simulink model "untitled"  (R2022a)
settings: Solver=FixedStepAuto  StartTime=0.0  StopTime=40  FixedStep=0.001768  RelTol=1e-3  EnableMultiTasking=on
values from neighbouring files (symbols this model uses):
  AlphacKhwgr = 0    [MELMNNSTRCECP.m]
  AlphavKhwgr = 0.914    [MELMNNSTRCECP.m]
  gr = 4    [MELMNNSTRCECP.m]
  JrC1 = 0.0675    [MELMNNSTRCECP.m]
  Khw = 5.81    [MELMNNSTRCECP.m]
libraries: dspstat3 x1, spsTriangleGeneratorLib x1
settings Model: Creator=dimas  LastModifiedBy=dimas
settings DataIOCC: SaveFormat=Array  ReturnWorkspaceOutputs=off
settings DebuggingCC: SolverPrmCheckMsg=warning  UnconnectedInputMsg=warning  UnconnectedOutputMsg=warning  UnconnectedLineMsg=warning  SFUnexpectedBacktrackingDiag=warning  SFNoUnconditionalDefaultTransitionDiag=warning  SFExecutionAtInitializationDiag=none  UnderSpecifiedDimensionMsg=warning
settings ModelReferenceCC: PropagateSignalLabelsOutOfModel=off
settings CodeAppCC: StateflowObjectComments=on
settings GRTTargetCC: TargetLangStandard=C89/C90 (ANSI)

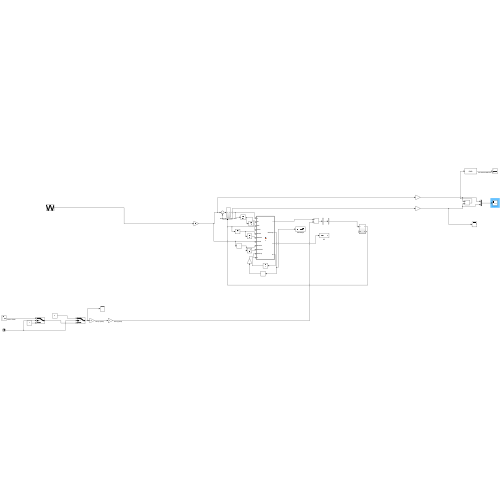
[thumbnail: Simulink's stored preview of the top-level diagram]
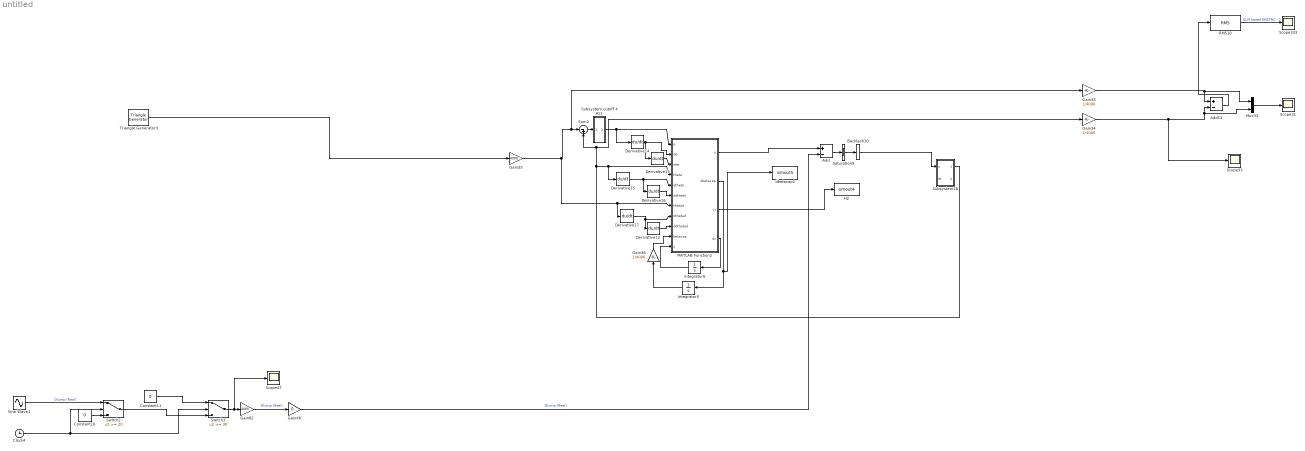
== system untitled ==
  Add : Sum  Inputs=+-
  Add11 : Sum  Inputs=+-
  Backlash10 : Backlash  BacklashWidth=BACKLASH
  Clock4 : Clock
  Constant10 : Constant  Value=0
  Constant11 : Constant  Value=0
  Derivative{12..17} (6 alike) : Derivative
  Gain33 : Gain  Gain=1/4000
  Gain34 : Gain  Gain=1/4000
  Gain35 : Gain  Gain=4000
  Gain36 : Gain  Gain=1/4000
  Gain48 : Gain  Gain=0
  Gain82 : Gain  Gain=4000
  H2 : ToWorkspace  VariableName=simout4  SaveFormat=Timeseries  SampleTime=-1
  Integrator5 : Integrator
  Integrator6 : Integrator
  MATLAB Function2 : MATLAB Function  TreatAsAtomicUnit=on
  Mux33 : Mux  Inputs=2
  RMS10 : dspstat3/RMS  run=off  directionMode=Each column  dimension=1  InputProcessing=Columns as channels (frame based)  reset_popup=None
  Saturation9 : Saturate  UpperLimit=32000  LowerLimit=-32000
  Scope{31,33,47,333} (4 alike) : Scope
  Sine Wave1 : Sin  Frequency=2*pi*0.2762  SampleTime=0.001768
  Subsystem cutoff 4 Hz1 : Subsystem
  Subsystem18 : Subsystem
  Sum2 : Sum  Inputs=|-+
  Switch2 : Switch  Threshold=20  SaturateOnIntegerOverflow=off  InputSameDT=off
  Switch3 : Switch  Threshold=30  SaturateOnIntegerOverflow=off  InputSameDT=off
  Triangle Generator3 : spsTriangleGeneratorLib/Triangle Generator  Freq=0.2762  Phase=180  Ts=0.001768
  dbetacap2 : ToWorkspace  VariableName=simout5  SaveFormat=Timeseries  SampleTime=-1
  wires:
  Gain36/1 -> MATLAB Function2/10(betacap)
  Integrator5/1 -> Gain36/1
  Add/1 -> Saturation9/1
  Derivative12/1 -> MATLAB Function2/9(ddthetad)
  Derivative13/1 -> MATLAB Function2/3(dde)
  Saturation9/1 -> Backlash10/1
  MATLAB Function2/3(H) -> H2/1
  MATLAB Function2/2(dbetacap) -> Integrator5/1, dbetacap2/1
  Gain34/1 -> Scope33/1, Add11/2, Mux33/2
  MATLAB Function2/4(dz) -> Integrator6/1
  Integrator6/1 -> MATLAB Function2/11(z)
  Derivative17/1 -> MATLAB Function2/8(dthetad), Derivative12/1
  Derivative14/1 -> MATLAB Function2/2(de), Derivative13/1
  Gain33/1 -> Add11/1, Mux33/1
  Sum2/1 -> Subsystem cutoff 4 Hz1/1(In1)
  Mux33/1 -> Scope31/1
  Subsystem18/1(Out1) -> Gain34/1, Sum2/2, MATLAB Function2/4(theta), Derivative15/1
  Add11/1 -> RMS10/1
  Gain35/1 -> Derivative17/1, MATLAB Function2/7(thetad), Gain33/1, Sum2/1
  Derivative16/1 -> MATLAB Function2/6(ddtheta)
  Derivative15/1 -> Derivative16/1, MATLAB Function2/5(dtheta)
  Backlash10/1 -> Subsystem18/1(u)
  MATLAB Function2/1(u) -> Add/1
  Subsystem cutoff 4 Hz1/1(Out1) -> MATLAB Function2/1(e), Derivative14/1
  Sine Wave1/1 -> Switch2/1  "Dlump (Real)"
  Gain48/1 -> Add/2  "Dlump (Real)"
  Gain82/1 -> Gain48/1  "Dlump (Real)"
  Constant11/1 -> Switch3/1
  Clock4/1 -> Switch3/2, Switch2/2
  Switch3/1 -> Scope47/1, Gain82/1
  Constant10/1 -> Switch2/3
  Switch2/1 -> Switch3/3
  Triangle Generator3/1 -> Gain35/1
  RMS10/1 -> Scope333/1  "ELM based NNSTRC - 2"

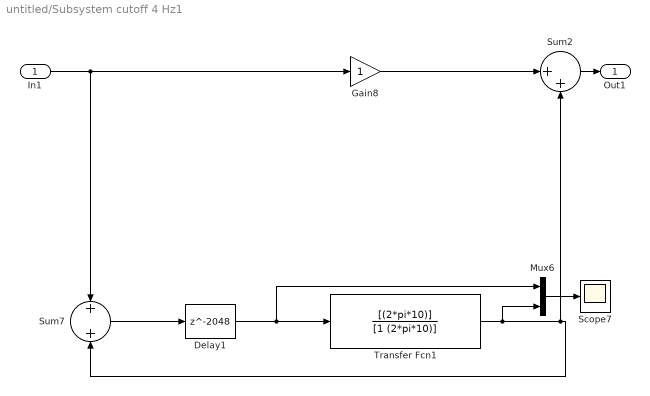
== system untitled/Subsystem cutoff 4 Hz1 ==
  In1 : Inport
  Delay1 : Delay  DelayLength=2048  SampleTime=0.001768
  Gain8 : Gain
  Mux6 : Mux  Inputs=2
  Scope7 : Scope
  Sum2 : Sum  Inputs=|++  InputSameDT=on  SaturateOnIntegerOverflow=on  OutDataTypeStr=Inherit: Same as first input
  Sum7 : Sum  Inputs=+|+  InputSameDT=on  SaturateOnIntegerOverflow=on  OutDataTypeStr=Inherit: Same as first input
  Transfer Fcn1 : TransferFcn  Numerator=[(2*pi*10)]  Denominator=[1 (2*pi*10)]
  Out1 : Outport  VectorParamsAs1DForOutWhenUnconnected=off
  wires:
  Gain8/1 -> Sum2/1
  Delay1/1 -> Transfer Fcn1/1, Mux6/1
  Mux6/1 -> Scope7/1
  Sum7/1 -> Delay1/1
  In1/1 -> Gain8/1, Sum7/1
  Sum2/1 -> Out1/1
  Transfer Fcn1/1 -> Mux6/2, Sum2/2, Sum7/2

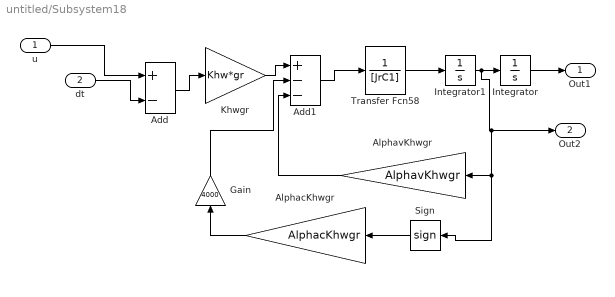
== system untitled/Subsystem18 ==
  u : Inport
  dt : Inport  Port=2
  Add : Sum  Inputs=+-
  Add1 : Sum  Inputs=+--
  AlphacKhwgr : Gain  Gain=AlphacKhwgr
  AlphavKhwgr : Gain  Gain=AlphavKhwgr
  Gain : Gain  Gain=4000
  Integrator : Integrator
  Integrator1 : Integrator
  Khwgr : Gain  Gain=Khw*gr
  Sign : Signum
  Transfer Fcn58 : TransferFcn  Denominator=[JrC1]
  Out1 : Outport  VectorParamsAs1DForOutWhenUnconnected=off
  Out2 : Outport  Port=2  VectorParamsAs1DForOutWhenUnconnected=off
  wires:
  u/1 -> Add/1
  Integrator/1 -> Out1/1
  dt/1 -> Add/2
  Add/1 -> Khwgr/1
  Add1/1 -> Transfer Fcn58/1
  Sign/1 -> AlphacKhwgr/1
  Integrator1/1 -> Sign/1, AlphavKhwgr/1, Out2/1, Integrator/1
  AlphavKhwgr/1 -> Add1/3
  Transfer Fcn58/1 -> Integrator1/1
  Khwgr/1 -> Add1/1
  AlphacKhwgr/1 -> Gain/1
  Gain/1 -> Add1/2

== matlab function untitled/MATLAB Function2 ==
  settings: updateMethod=DISCRETE
  data: e input; de input; dde input; u output; theta input; dtheta input; ddtheta input; thetad input; dthetad input; ddthetad input; betacap input; dbetacap output; H output; z input; dz output
function [u,dbetacap,H,dz]   = fcn(e,de,dde,theta,dtheta,ddtheta,thetad,dthetad,ddthetad,betacap,z)

JrC1=0.0675;
Khw=5.81;
gr=4;
AlphavKhwgr=0.914;
AlphacKhwgr=0;

b0=Khw*gr;
Beq0=AlphavKhwgr;
Jeq0=JrC1;
Fs0=AlphacKhwgr;
TLH0=0.3193;
ksp0=0.0914;
theta0=12/180*pi;

k1=0.1;
k2=0.5;
k3=0.1;
kp=-5;
ki=-20;
kd=-0.5;
%miu1=0.002;
miu1=200/10;
%miu2=200;
miu2=200/10;

geta1=9/7;
geta2=17/9;
geta3=9/7;
delta=0.1;
n=200;
delN=25;
rol=20;



%gamaij=[-1 -11/12 -10/12 -9/12 -8/12 -7/12 -6/12 -5/12 -4/12 -3/12 -2/12 -1/12 0 1/12 2/12 3/12 4/12 5/12 6/12 7/12 8/12 9/12 10/12 11/12 1];
gamaij=-1 + (1+1)*rand(3,25);
alphaj=rand(1,25);

x1=theta;
x2=dtheta;
x3=ddtheta;
xi=[x1 x2 x3];

H=zeros(1,delN);
betacap1=zeros(1,delN); %[betacap(1) betacap(2) betacap(3) betacap(4) betacap(5) betacap(6) betacap(7) betacap(8) betacap(9) betacap(10) betacap(11) betacap(12) betacap(13) betacap(14) betacap(15) betacap(16) betacap(17) betacap(18) betacap(19) betacap(20) betacap(21) betacap(22) betacap(23) betacap(24) betacap(25)];


for j=1:1:delN
H(j)=1/(1+exp(-((xi*gamaij(:,j))+alphaj(j))));
end

for j=1:1:delN
betacap1(j)=betacap(j);
end

dcaplump=H*betacap1.';

c=50/10;

%s=e+k1*((abs(de))^(geta1))*sign(de)+k2*((abs(e))^(geta2))*sign(e);

s=de+c*e;

dD=0.10*4000;
miu11=25/10000; %1.5

%miu22=1581.1; %1.5
miu22=10/10000;

landa11=miu22*sqrt(dD);
landa22=miu11*dD;
dz=landa22*sign(s);
%u0=-landa11*sqrt(abs(s))*sign(s)-z+ddthetad-c*de; 

dbetacap=n*k1*geta1*((abs(de))^(geta1-1))*(abs(s))*H;

Tfsp0=Fs0*sign(dtheta)+TLH0*sign(theta-theta0);
%u0=(Jeq0/b0)*(-landa11*sqrt(abs(s))*sign(s)-z+ddthetad-c*de);

%u0=-((Jeq0)/(b0*k1*geta1))*((abs(de))^(2-geta1))*sign(de)-((Jeq0*k2*geta2)/(b0*k1*geta1))*((abs(e))^(geta2-1))*((abs(de))^(2-geta2))*sign(de)+(Beq0/b0)*dtheta+(Tfsp0/b0)+(Jeq0/b0)*(ddthetad);

%u1=-(Jeq0/b0)*dcaplump*sign(s);

%u2=-(Jeq0/b0)*(miu1*sign(s)+miu2*s);

u1=-(1/b0)*dcaplump*sign(s);

u2=-(1/b0)*(1/Tfsp0+c*de+c*s);    

u=u1+u2;
